simulink model "problem1_block_cl"  (R2024b)
settings: Solver=ode4  StartTime=0.0  StopTime=10  FixedStep=9.4596e-05  RelTol=1e-3
values from neighbouring files (symbols this model uses):
  A_c = pi * D_c^2 / 4    (= 0.00196349540849)    [problem1.m]    (also in problem2.m = w * t; problem3.m = w * t)
  b = 1800    [problem1.m]    (also in problem2.m = feasible(1,:); problem3.m = feasible(1,:))
  k_cyl = 9.0e4    (= 90000)    [problem1.m]
  m = 1200    [problem1.m]    (also in problem2.m = sqrt((P / A_c) * (h / k_fin)); problem3.m = sqrt((P / A_c) * (h / k_fin)))
  P_s = 13.8e6    (= 13800000)    [problem1.m]
  Q_max = 2.5e-4    (= 0.00025)    [problem1.m]
  tau_v = 0.03    [problem1.m]
undefined symbols (not defined in the file or in its folder): den_cl, num_cl
settings Model: Creator=piero  LastModifiedBy=piero

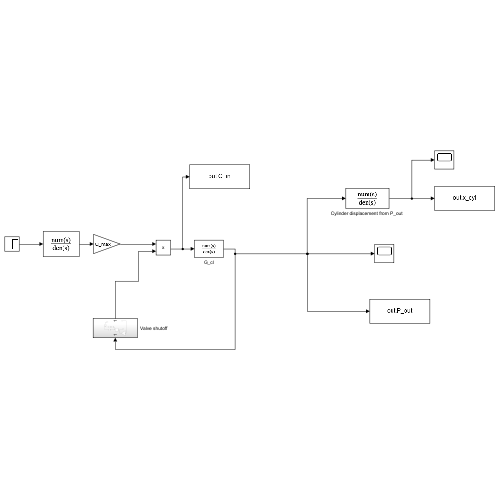
[thumbnail: Simulink's stored preview of the top-level diagram]
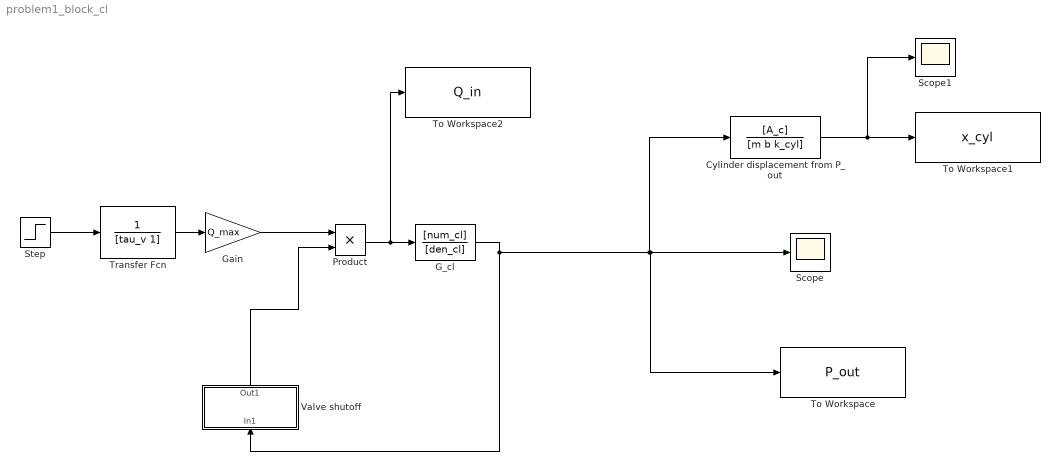
== system problem1_block_cl ==
  "Cylinder displacement from P_out " : TransferFcn  Numerator=[A_c]  Denominator=[m b k_cyl]
  G_cl : TransferFcn  Numerator=[num_cl]  Denominator=[den_cl]
  Gain : Gain  Gain=Q_max
  Product : Product
  Scope : Scope
  Scope1 : Scope
  Step : Step  Time=0  SampleTime=0
  To Workspace : ToWorkspace  VariableName=P_out  SaveFormat=Timeseries  SampleTime=-1
  To Workspace1 : ToWorkspace  VariableName=x_cyl  SaveFormat=Timeseries  SampleTime=-1
  To Workspace2 : ToWorkspace  VariableName=Q_in  SaveFormat=Timeseries  SampleTime=-1
  Transfer Fcn : TransferFcn  Denominator=[tau_v 1]
  "Valve shutoff " : Subsystem
  wires:
  "Cylinder displacement from P_out "/1 -> To Workspace1/1, Scope1/1
  "Valve shutoff "/1(Out1) -> Product/2
  Product/1 -> G_cl/1, To Workspace2/1
  Gain/1 -> Product/1
  Transfer Fcn/1 -> Gain/1
  Step/1 -> Transfer Fcn/1
  G_cl/1 -> "Cylinder displacement from P_out "/1, To Workspace/1, Scope/1, "Valve shutoff "/1(In1)

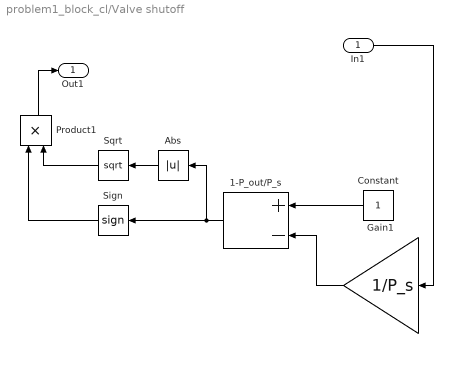
== system problem1_block_cl/Valve shutoff  ==
  In1 : Inport
  1-P_out/P_s : Sum  Inputs=+-
  Abs : Abs  SaturateOnIntegerOverflow=off
  Constant : Constant
  Gain1 : Gain  Gain=1/P_s
  Product1 : Product
  Sign : Signum
  Sqrt : Sqrt
  Out1 : Outport
  wires:
  Constant/1 -> 1-P_out/P_s/1
  1-P_out/P_s/1 -> Sign/1, Abs/1
  Gain1/1 -> 1-P_out/P_s/2
  Sqrt/1 -> Product1/2
  Abs/1 -> Sqrt/1
  Sign/1 -> Product1/1
  In1/1 -> Gain1/1
  Product1/1 -> Out1/1
